simulink model "VB_RIFKF_UWB_INS25"  (R2023a)
settings: Solver=FixedStepAuto  StartTime=0.0  StopTime=500  FixedStep=0.01  RelTol=1e-3
InitFcn:
  | resilient_initNavigation1216;
  | init_param;
  | param_bias;
undefined symbols (not defined in the file or in its folder): dt, g0, gam0_rad, ISUS_flag, lp_GPS_sample_time, lp_Lidar_knoise, lp_Lidar_max, lp_Lidar_min, lp_Lidar_sample_time, lp_Lidar_seed, lp_UWB_knoise, lp_UWB_sample_time, lp_UWB_seed, lp_UWB_XY_max, lp_UWB_XY_min, magnitude, p, P0, P0_RIEKF, param, pd0, pe0, phi0_rad, pn0, psi, psi0_rad, state_dim, vd0, ve0, vn0
libraries: simulink_extras x108, simulink x89, dspstat3 x74, sharedtransform x61, matrix_library x11, sharedTrackingLibrary x8, aerolibconvert2 x5, aerolibtransform2 x5, dspfactors x3
(part 2 of 29)

== system VB_RIFKF_UWB_INS25/read FC1_zy ==
  Bus Creator : BusCreator  Inputs=3
  Bus Creator1 : BusCreator  Inputs=3
  Bus Creator2 : BusCreator  Inputs=3
  Degrees to Radians : simulink_extras/Transformations/Degrees to Radians
  Degrees to Radians1 : simulink_extras/Transformations/Degrees to Radians
  Degrees to Radians2 : simulink_extras/Transformations/Degrees to Radians
  From Workspace1 : FromWorkspace  VariableName=[time(1:(end-1)),FCS1.data_tj_st.Vn(1:(end-1))]
  From Workspace10 : FromWorkspace  VariableName=[time(1:(end-1)),FCS1.data_tj_st.Ve(1:(end-1))]
  From Workspace11 : FromWorkspace  VariableName=[time(1:(end-1)),FCS1.data_tj_st.Vu(1:(end-1))]
  From Workspace12 : FromWorkspace  VariableName=[time(1:(end-1)),FCS1.data_zy_st.gy(1:(end-1))]
  From Workspace13 : FromWorkspace  VariableName=[time(1:(end-1)),FCS1.data_zy_st.gz(1:(end-1))]
  From Workspace14 : FromWorkspace  VariableName=[time(1:(end-1)),FCS1.data_zy_st.Ax(1:(end-1))]
  From Workspace15 : FromWorkspace  VariableName=[time(1:(end-1)),FCS1.data_zy_st.Ay(1:(end-1))]
  From Workspace16 : FromWorkspace  VariableName=[time(1:(end-1)),FCS1.data_zy_st.Az(1:(end-1))]
  From Workspace17 : FromWorkspace  VariableName=[time(1:(end-1)),FCS1.data_zy_st.roll(1:(end-1))]
  From Workspace18 : FromWorkspace  VariableName=[time(1:(end-1)),FCS1.data_zy_st.pitch(1:(end-1))]
  From Workspace19 : FromWorkspace  VariableName=[time(1:(end-1)),FCS1.data_zy_st.yaw(1:(end-1))]
  From Workspace2 : FromWorkspace  VariableName=[time(1:(end-1)),FCS1.data_zy_st.gx(1:(end-1))]
  From Workspace7 : FromWorkspace  VariableName=[time(1:(end-1)),FCS1.data_zy_st.lat(1:(end-1))]
  From Workspace8 : FromWorkspace  VariableName=[time(1:(end-1)),FCS1.data_zy_st.lon(1:(end-1))]
  From Workspace9 : FromWorkspace  VariableName=[time(1:(end-1)),FCS1.data_zy_st.height(1:(end-1))]
  Gain1 : Gain  Gain=-1
  MATLAB Function : MATLAB Function  TreatAsAtomicUnit=on
  Mux : Mux  Inputs=3
  Mux2 : Mux  Inputs=3
  Mux3 : Mux  Inputs=3
  Scope{,2,4..9} (8 alike) : Scope
  Subsystem : Subsystem
  Subsystem1 : Subsystem
  Subsystem2 : Subsystem
  Zero-Order Hold9 : ZeroOrderHold  SampleTime=dt
  vned_GPS : Outport
  GPS_lla_rad : Outport  Port=2
  wxyz : Outport  Port=3
  fbxyz : Outport  Port=4
  magn : Outport  Port=5
  att_ref : Outport  Port=6
  wires:
  Mux3/1 -> Zero-Order Hold9/1
  From Workspace17/1 -> Bus Creator2/1  "roll"
  From Workspace19/1 -> MATLAB Function/1(dpsi)
  From Workspace11/1 -> Gain1/1
  Bus Creator2/1 -> Scope9/1, att_ref/1, Scope8/1
  Degrees to Radians2/1 -> wxyz/1, Scope6/1
  From Workspace15/1 -> Bus Creator1/2
  Subsystem/1(y) -> Bus Creator/1
  From Workspace14/1 -> Bus Creator1/1
  Zero-Order Hold9/1 -> magn/1
  Degrees to Radians1/1 -> Mux2/2
  Subsystem2/1(y) -> Bus Creator/3
  MATLAB Function/1(y) -> Bus Creator2/3  "yaw"
  From Workspace1/1 -> Mux/1  "vn"
  From Workspace9/1 -> Mux2/3  "altitude"
  Mux/1 -> Scope2/1, vned_GPS/1
  From Workspace16/1 -> Bus Creator1/3
  From Workspace12/1 -> Scope7/1, Subsystem1/1(u)
  From Workspace8/1 -> Degrees to Radians1/1  "lon"
  Bus Creator/1 -> Scope4/1, Degrees to Radians2/1
  Bus Creator1/1 -> fbxyz/1, Scope5/1
  Mux2/1 -> GPS_lla_rad/1, Scope/1
  Gain1/1 -> Mux/3
  From Workspace18/1 -> Bus Creator2/2  "pitch"
  From Workspace10/1 -> Mux/2  "ve"
  Degrees to Radians/1 -> Mux2/1
  Subsystem1/1(y) -> Bus Creator/2
  From Workspace7/1 -> Degrees to Radians/1  "lat"
  From Workspace2/1 -> Subsystem/1(u)
  From Workspace13/1 -> Subsystem2/1(u)

== system VB_RIFKF_UWB_INS25/read FC1_zy1 ==
  Bus Creator2 : BusCreator  Inputs=3
  Degrees to Radians : simulink_extras/Transformations/Degrees to Radians
  Degrees to Radians1 : simulink_extras/Transformations/Degrees to Radians
  From Workspace1 : FromWorkspace  VariableName=[time(1:(end-1)),FCS1.data_tj_st.Vn(1:(end-1))]
  From Workspace10 : FromWorkspace  VariableName=[time(1:(end-1)),FCS1.data_tj_st.Ve(1:(end-1))]
  From Workspace11 : FromWorkspace  VariableName=[time(1:(end-1)),FCS1.data_tj_st.Vu(1:(end-1))]
  From Workspace17 : FromWorkspace  VariableName=[time(1:(end-1)),FCS1.data_zy_st.roll(1:(end-1))]
  From Workspace18 : FromWorkspace  VariableName=[time(1:(end-1)),FCS1.data_zy_st.pitch(1:(end-1))]
  From Workspace19 : FromWorkspace  VariableName=[time(1:(end-1)),FCS1.data_zy_st.yaw(1:(end-1))]
  From Workspace7 : FromWorkspace  VariableName=[time(1:(end-1)),FCS1.data_tj_st.lat(1:(end-1))]
  From Workspace8 : FromWorkspace  VariableName=[time(1:(end-1)),FCS1.data_tj_st.lon(1:(end-1))]
  From Workspace9 : FromWorkspace  VariableName=[time(1:(end-1)),FCS1.data_tj_st.height(1:(end-1))]
  Gain1 : Gain  Gain=-1
  MATLAB Function : MATLAB Function  TreatAsAtomicUnit=on
  Mux : Mux  Inputs=3
  Mux2 : Mux  Inputs=3
  Mux3 : Mux  Inputs=3
  Scope{,2,8..9} (4 alike) : Scope
  Zero-Order Hold9 : ZeroOrderHold  SampleTime=dt
  vned_GPS : Outport
  GPS_lla_rad : Outport  Port=2
  magn : Outport  Port=3
  att_ref : Outport  Port=4
  wires:
  From Workspace7/1 -> Degrees to Radians/1  "lat"
  Degrees to Radians/1 -> Mux2/1
  From Workspace10/1 -> Mux/2  "ve"
  From Workspace18/1 -> Bus Creator2/2  "pitch"
  Gain1/1 -> Mux/3
  Mux2/1 -> Scope/1, GPS_lla_rad/1
  From Workspace8/1 -> Degrees to Radians1/1  "lon"
  Mux/1 -> vned_GPS/1, Scope2/1
  From Workspace9/1 -> Mux2/3  "altitude"
  From Workspace1/1 -> Mux/1  "vn"
  MATLAB Function/1(y) -> Bus Creator2/3  "yaw"
  Degrees to Radians1/1 -> Mux2/2
  Zero-Order Hold9/1 -> magn/1
  Bus Creator2/1 -> Scope8/1, att_ref/1, Scope9/1
  From Workspace11/1 -> Gain1/1
  From Workspace19/1 -> MATLAB Function/1(dpsi)
  From Workspace17/1 -> Bus Creator2/1  "roll"
  Mux3/1 -> Zero-Order Hold9/1

== system VB_RIFKF_UWB_INS25/read FC6_zy2 ==
  Bus Creator : BusCreator  Inputs=3
  Bus Creator1 : BusCreator  Inputs=3
  Bus Creator2 : BusCreator  Inputs=3
  Degrees to Radians : simulink_extras/Transformations/Degrees to Radians
  Degrees to Radians1 : simulink_extras/Transformations/Degrees to Radians
  Degrees to Radians2 : simulink_extras/Transformations/Degrees to Radians
  From Workspace1 : FromWorkspace  VariableName=[time1(1:(end-1)),FCS6.data_zy_st.Vn(1:(end-1))]
  From Workspace10 : FromWorkspace  VariableName=[time1(1:(end-1)),FCS6.data_zy_st.Ve(1:(end-1))]
  From Workspace11 : FromWorkspace  VariableName=[time1(1:(end-1)),FCS6.data_zy_st.Vu(1:(end-1))]
  From Workspace12 : FromWorkspace  VariableName=[time1(1:(end-1)),FCS6.data_hf_st.gy(1:(end-1))]
  From Workspace13 : FromWorkspace  VariableName=[time1(1:(end-1)),FCS6.data_hf_st.gz(1:(end-1))]
  From Workspace14 : FromWorkspace  VariableName=[time1(1:(end-1)),FCS6.data_hf_st.Ax(1:(end-1))]
  From Workspace15 : FromWorkspace  VariableName=[time1(1:(end-1)),FCS6.data_hf_st.Ay(1:(end-1))]
  From Workspace16 : FromWorkspace  VariableName=[time1(1:(end-1)),FCS6.data_hf_st.Az(1:(end-1))]
  From Workspace17 : FromWorkspace  VariableName=[time1(1:(end-1)),FCS6.data_zy_st.roll(1:(end-1))]
  From Workspace18 : FromWorkspace  VariableName=[time1(1:(end-1)),FCS6.data_zy_st.pitch(1:(end-1))]
  From Workspace19 : FromWorkspace  VariableName=[time1(1:(end-1)),FCS6.data_zy_st.yaw(1:(end-1))]
  From Workspace2 : FromWorkspace  VariableName=[time1(1:(end-1)),FCS6.data_hf_st.gx(1:(end-1))]
  From Workspace7 : FromWorkspace  VariableName=[time1(1:(end-1)),FCS6.data_zy_st.lat(1:(end-1))]
  From Workspace8 : FromWorkspace  VariableName=[time1(1:(end-1)),FCS6.data_zy_st.lon(1:(end-1))]
  From Workspace9 : FromWorkspace  VariableName=[time1(1:(end-1)),FCS6.data_zy_st.height(1:(end-1))]
  Gain1 : Gain  Gain=-1
  MATLAB Function : MATLAB Function  TreatAsAtomicUnit=on
  Mux : Mux  Inputs=3
  Mux2 : Mux  Inputs=3
  Mux3 : Mux  Inputs=3
  Scope{,2,4..6,8..9} (7 alike) : Scope
  Subsystem : Subsystem
  Subsystem1 : Subsystem
  Subsystem2 : Subsystem
  Zero-Order Hold9 : ZeroOrderHold  SampleTime=dt
  wxyz : Outport
  fbxyz : Outport  Port=2
  vned_GPS : Outport  Port=3
  GPS_lla_rad : Outport  Port=4
  magn : Outport  Port=5
  att_ref : Outport  Port=6
  wires:
  Mux3/1 -> Zero-Order Hold9/1
  From Workspace17/1 -> Bus Creator2/1  "roll"
  From Workspace19/1 -> MATLAB Function/1(dpsi)
  From Workspace11/1 -> Gain1/1
  Bus Creator2/1 -> Scope9/1, att_ref/1, Scope8/1
  Zero-Order Hold9/1 -> magn/1
  Degrees to Radians1/1 -> Mux2/2
  MATLAB Function/1(y) -> Bus Creator2/3  "yaw"
  From Workspace1/1 -> Mux/1  "vn"
  From Workspace9/1 -> Mux2/3  "altitude"
  Mux/1 -> Scope2/1, vned_GPS/1
  From Workspace8/1 -> Degrees to Radians1/1  "lon"
  Mux2/1 -> GPS_lla_rad/1, Scope/1
  Gain1/1 -> Mux/3
  From Workspace18/1 -> Bus Creator2/2  "pitch"
  From Workspace10/1 -> Mux/2  "ve"
  Degrees to Radians/1 -> Mux2/1
  From Workspace7/1 -> Degrees to Radians/1  "lat"
  From Workspace2/1 -> Subsystem/1(u)
  Subsystem1/1(y) -> Bus Creator/2
  From Workspace13/1 -> Subsystem2/1(u)
  Bus Creator1/1 -> fbxyz/1, Scope5/1
  Degrees to Radians2/1 -> wxyz/1, Scope6/1
  Subsystem2/1(y) -> Bus Creator/3
  From Workspace15/1 -> Bus Creator1/2
  Subsystem/1(y) -> Bus Creator/1
  From Workspace16/1 -> Bus Creator1/3
  Bus Creator/1 -> Scope4/1, Degrees to Radians2/1
  From Workspace12/1 -> Subsystem1/1(u)
  From Workspace14/1 -> Bus Creator1/1

== system VB_RIFKF_UWB_INS25/相对传感器模拟1 ==
  #2P : Inport
  #1GPS1 : Inport  Port=2
  Add : Sum  Inputs=-+
  Add2 : Sum  Inputs=+-
  Atan1 : Trigonometry  Operator=atan2
  Atan3 : Trigonometry  Operator=cos
  Atan4 : Trigonometry
  Bus Creator : BusCreator  Inputs=5
  Bus Selector : BusSelector  OutputSignals=GPS_Data.pos_N_gps,GPS_Data.pos_E_gps,GPS_Data.pos_D_gps
  Bus Selector1 : BusSelector  OutputSignals=GPS_Data.pos_N_gps,GPS_Data.pos_E_gps,GPS_Data.pos_D_gps
  Delay : Delay  DelayLength=1
  Delay1 : Delay  DelayLength=1
  Delay2 : Delay  DelayLength=1
  Display : Display
  Display2 : Display
  Display3 : Display
  Dot Product : DotProduct  OutDataTypeStr=Inherit: Inherit via internal rule
  MATLAB Function : MATLAB Function  Commented=on  TreatAsAtomicUnit=on
  Mux : Mux  Inputs=2
  Mux1 : Mux  Inputs=3
  Mux2 : Mux  Inputs=2
  Mux3 : Mux  Inputs=3
  Radians to Degrees1 : simulink_extras/Transformations/Radians to Degrees
  Radians to Degrees2 : simulink_extras/Transformations/Radians to Degrees
  Radians to Degrees3 : simulink_extras/Transformations/Radians to Degrees
  Scope{,1..2,4,6..9} (8 alike) : Scope
  Scope10 : Scope  NumInputPorts=2
  Sqrt3 : Sqrt
  Subsystem : Subsystem
  Subsystem2 : Subsystem
  Sum of Elements : Sum  Inputs=+
  delta_x : Selector  InputPortWidth=3  IndexOptions=Index vector (dialog)  Indices=[1]  OutputSizes=1
  delta_x2 : Selector  InputPortWidth=3  IndexOptions=Index vector (dialog)  Indices=[1 2]  OutputSizes=1
  delta_y : Selector  InputPortWidth=3  IndexOptions=Index vector (dialog)  Indices=[2]  OutputSizes=1
  p_r_psi_phi : Outport
  wires:
  #1GPS1/1 -> Bus Selector/1
  Delay2/1 -> Bus Creator/4  "p2_k-1"
  Delay1/1 -> Mux2/2
  Delay/1 -> Mux/2
  #2P/1 -> Bus Selector1/1  "p2"
  Bus Selector1/3 -> Mux3/3  "<pos_D_gps>"
  Bus Selector1/2 -> Mux3/2  "<pos_E_gps>"
  Bus Selector1/1 -> Mux3/1  "<pos_N_gps>"
  Bus Selector/3 -> Mux1/3  "<pos_D_gps>"
  Bus Selector/2 -> Mux1/2  "<pos_E_gps>"
  Bus Selector/1 -> Mux1/1  "<pos_N_gps>"
  Add2/1 -> Scope8/1
  Atan1/1 -> Mux/1, Atan3/1, Atan4/1, Radians to Degrees2/1, Delay/1
  Mux3/1 -> Add/2, Scope10/2, Bus Creator/3, Delay2/1  "p2"
  Atan4/1 -> Scope7/1
  Atan3/1 -> Scope6/1
  MATLAB Function/1(y) -> Radians to Degrees3/1
  Radians to Degrees3/1 -> Scope2/1
  delta_x2/1 -> Dot Product/2, Dot Product/1
  Radians to Degrees1/1 -> Scope1/1, Add2/2
  Mux1/1 -> Add/1, Scope10/1
  delta_x/1 -> Display3/1, MATLAB Function/2(dx), Atan1/2
  delta_y/1 -> Display2/1, MATLAB Function/1(dy), Atan1/1
  Mux/1 -> Subsystem/1("psi ")
  Mux2/1 -> Subsystem2/1(r_xyz)
  Sum of Elements/1 -> Sqrt3/1
  Dot Product/1 -> Sum of Elements/1
  Sqrt3/1 -> Mux2/1, Scope4/1, Delay1/1, Display/1  "r12"
  Subsystem2/1(r_xyz out) -> Bus Creator/2  "r"
  Add/1 -> delta_x2/1, delta_x/1, delta_y/1, Bus Creator/5, Scope9/1  "dp"
  Subsystem/1(psi  out) -> Bus Creator/1  "psi"
  Bus Creator/1 -> p_r_psi_phi/1
  Radians to Degrees2/1 -> Scope/1, Add2/1

== system VB_RIFKF_UWB_INS25/相对传感器模拟2 ==
  #2P : Inport
  #1GPS1 : Inport  Port=2
  #1GPS2 : Inport  Port=3
  Add : Sum  Inputs=-+
  Add2 : Sum  Inputs=+-
  Atan1 : Trigonometry  Operator=atan2
  Atan3 : Trigonometry  Operator=cos
  Atan4 : Trigonometry
  Bus Creator : BusCreator  Inputs=5
  Bus Selector : BusSelector  OutputSignals=GPS_Data.pos_N_gps,GPS_Data.pos_E_gps,GPS_Data.pos_D_gps
  Bus Selector1 : BusSelector  OutputSignals=GPS_Data.pos_N_gps,GPS_Data.pos_E_gps,GPS_Data.pos_D_gps
  Delay : Delay  DelayLength=1
  Delay1 : Delay  DelayLength=1
  Delay2 : Delay  DelayLength=1
  Digital Clock : DigitalClock  SampleTime=0.01
  Display : Display
  Display2 : Display
  Display3 : Display
  Dot Product : DotProduct  OutDataTypeStr=Inherit: Inherit via internal rule
  MATLAB Function : MATLAB Function  Commented=on  TreatAsAtomicUnit=on
  Mux : Mux  Inputs=2
  Mux1 : Mux  Inputs=3
  Mux2 : Mux  Inputs=2
  Mux3 : Mux  Inputs=3
  Radians to Degrees1 : simulink_extras/Transformations/Radians to Degrees
  Radians to Degrees2 : simulink_extras/Transformations/Radians to Degrees
  Radians to Degrees3 : simulink_extras/Transformations/Radians to Degrees
  Scope{,1..2,4,6..9} (8 alike) : Scope
  Scope10 : Scope  NumInputPorts=2
  Sqrt3 : Sqrt
  Subsystem : Subsystem
  Subsystem2 : Subsystem
  Sum of Elements : Sum  Inputs=+
  Switch2 : Switch  Criteria=u2 > Threshold  Threshold=300  SaturateOnIntegerOverflow=off  InputSameDT=off
  delta_x : Selector  InputPortWidth=3  IndexOptions=Index vector (dialog)  Indices=[1]  OutputSizes=1
  delta_x2 : Selector  InputPortWidth=3  IndexOptions=Index vector (dialog)  Indices=[1 2]  OutputSizes=1
  delta_y : Selector  InputPortWidth=3  IndexOptions=Index vector (dialog)  Indices=[2]  OutputSizes=1
  p_r_psi_phi : Outport
  wires:
  Radians to Degrees2/1 -> Add2/1, Scope/1
  Bus Creator/1 -> p_r_psi_phi/1
  Subsystem/1(psi  out) -> Bus Creator/1  "psi"
  Add/1 -> Scope9/1, Bus Creator/5, delta_y/1, delta_x/1, delta_x2/1  "dp"
  Subsystem2/1(r_xyz out) -> Bus Creator/2  "r"
  Sqrt3/1 -> Display/1, Delay1/1, Scope4/1, Mux2/1  "r12"
  Dot Product/1 -> Sum of Elements/1
  Sum of Elements/1 -> Sqrt3/1
  Mux2/1 -> Subsystem2/1(r_xyz)
  Mux/1 -> Subsystem/1("psi ")
  delta_y/1 -> Atan1/1, MATLAB Function/1(dy), Display2/1
  delta_x/1 -> Atan1/2, MATLAB Function/2(dx), Display3/1
  Mux1/1 -> Scope10/1, Add/1
  Radians to Degrees1/1 -> Add2/2, Scope1/1
  delta_x2/1 -> Dot Product/1, Dot Product/2
  Radians to Degrees3/1 -> Scope2/1
  MATLAB Function/1(y) -> Radians to Degrees3/1
  Atan3/1 -> Scope6/1
  Atan4/1 -> Scope7/1
  Mux3/1 -> Delay2/1, Bus Creator/3, Scope10/2, Add/2  "p2"
  Atan1/1 -> Delay/1, Radians to Degrees2/1, Atan4/1, Atan3/1, Mux/1
  Add2/1 -> Scope8/1
  #1GPS1/1 -> Switch2/3
  Bus Selector/1 -> Mux1/1  "<pos_N_gps>"
  Bus Selector/2 -> Mux1/2  "<pos_E_gps>"
  Bus Selector/3 -> Mux1/3  "<pos_D_gps>"
  Bus Selector1/1 -> Mux3/1  "<pos_N_gps>"
  Bus Selector1/2 -> Mux3/2  "<pos_E_gps>"
  Bus Selector1/3 -> Mux3/3  "<pos_D_gps>"
  #2P/1 -> Bus Selector1/1  "p2"
  Delay/1 -> Mux/2
  Delay1/1 -> Mux2/2
  Delay2/1 -> Bus Creator/4  "p2_k-1"
  Digital Clock/1 -> Switch2/2
  #1GPS2/1 -> Switch2/1
  Switch2/1 -> Bus Selector/1

== system VB_RIFKF_UWB_INS25/相对传感器模拟3 ==
  #2P : Inport
  #1GPS2 : Inport  Port=2
  Add : Sum  Inputs=-+
  Add2 : Sum  Inputs=+-
  Atan1 : Trigonometry  Operator=atan2
  Atan3 : Trigonometry  Operator=cos
  Atan4 : Trigonometry
  Bus Creator : BusCreator  Inputs=5
  Bus Selector : BusSelector  OutputSignals=GPS_Data.pos_N_gps,GPS_Data.pos_E_gps,GPS_Data.pos_D_gps
  Bus Selector1 : BusSelector  OutputSignals=GPS_Data.pos_N_gps,GPS_Data.pos_E_gps,GPS_Data.pos_D_gps
  Delay : Delay  DelayLength=1
  Delay1 : Delay  DelayLength=1
  Delay2 : Delay  DelayLength=1
  Display : Display
  Display2 : Display
  Display3 : Display
  Dot Product : DotProduct  OutDataTypeStr=Inherit: Inherit via internal rule
  MATLAB Function : MATLAB Function  Commented=on  TreatAsAtomicUnit=on
  Mux : Mux  Inputs=2
  Mux1 : Mux  Inputs=3
  Mux2 : Mux  Inputs=2
  Mux3 : Mux  Inputs=3
  Radians to Degrees1 : simulink_extras/Transformations/Radians to Degrees
  Radians to Degrees2 : simulink_extras/Transformations/Radians to Degrees
  Radians to Degrees3 : simulink_extras/Transformations/Radians to Degrees
  Scope{,1..2,4,6..9} (8 alike) : Scope
  Scope10 : Scope  NumInputPorts=2
  Sqrt3 : Sqrt
  Subsystem : Subsystem
  Subsystem2 : Subsystem
  Sum of Elements : Sum  Inputs=+
  delta_x : Selector  InputPortWidth=3  IndexOptions=Index vector (dialog)  Indices=[1]  OutputSizes=1
  delta_x2 : Selector  InputPortWidth=3  IndexOptions=Index vector (dialog)  Indices=[1 2]  OutputSizes=1
  delta_y : Selector  InputPortWidth=3  IndexOptions=Index vector (dialog)  Indices=[2]  OutputSizes=1
  p_r_psi_phi : Outport
  wires:
  Radians to Degrees2/1 -> Add2/1, Scope/1
  Bus Creator/1 -> p_r_psi_phi/1
  Subsystem/1(psi  out) -> Bus Creator/1  "psi"
  Add/1 -> Scope9/1, Bus Creator/5, delta_y/1, delta_x/1, delta_x2/1  "dp"
  Subsystem2/1(r_xyz out) -> Bus Creator/2  "r"
  Sqrt3/1 -> Display/1, Delay1/1, Scope4/1, Mux2/1  "r12"
  Dot Product/1 -> Sum of Elements/1
  Sum of Elements/1 -> Sqrt3/1
  Mux2/1 -> Subsystem2/1(r_xyz)
  Mux/1 -> Subsystem/1("psi ")
  delta_y/1 -> Atan1/1, MATLAB Function/1(dy), Display2/1
  delta_x/1 -> Atan1/2, MATLAB Function/2(dx), Display3/1
  Mux1/1 -> Scope10/1, Add/1
  Radians to Degrees1/1 -> Add2/2, Scope1/1
  delta_x2/1 -> Dot Product/1, Dot Product/2
  Radians to Degrees3/1 -> Scope2/1
  MATLAB Function/1(y) -> Radians to Degrees3/1
  Atan3/1 -> Scope6/1
  Atan4/1 -> Scope7/1
  Mux3/1 -> Delay2/1, Bus Creator/3, Scope10/2, Add/2  "p2"
  Atan1/1 -> Delay/1, Radians to Degrees2/1, Atan4/1, Atan3/1, Mux/1
  Add2/1 -> Scope8/1
  Bus Selector/1 -> Mux1/1  "<pos_N_gps>"
  Bus Selector/2 -> Mux1/2  "<pos_E_gps>"
  Bus Selector/3 -> Mux1/3  "<pos_D_gps>"
  Bus Selector1/1 -> Mux3/1  "<pos_N_gps>"
  Bus Selector1/2 -> Mux3/2  "<pos_E_gps>"
  Bus Selector1/3 -> Mux3/3  "<pos_D_gps>"
  #2P/1 -> Bus Selector1/1  "p2"
  Delay/1 -> Mux/2
  Delay1/1 -> Mux2/2
  Delay2/1 -> Bus Creator/4  "p2_k-1"
  #1GPS2/1 -> Bus Selector/1

== system VB_RIFKF_UWB_INS25/相对传感器模拟4 ==
  #2P : Inport
  #1GPS3 : Inport  Port=2
  Add : Sum  Inputs=-+
  Add2 : Sum  Inputs=+-
  Atan1 : Trigonometry  Operator=atan2
  Atan3 : Trigonometry  Operator=cos
  Atan4 : Trigonometry
  Bus Creator : BusCreator  Inputs=5
  Bus Selector : BusSelector  OutputSignals=GPS_Data.pos_N_gps,GPS_Data.pos_E_gps,GPS_Data.pos_D_gps
  Bus Selector1 : BusSelector  OutputSignals=GPS_Data.pos_N_gps,GPS_Data.pos_E_gps,GPS_Data.pos_D_gps
  Delay : Delay  DelayLength=1
  Delay1 : Delay  DelayLength=1
  Delay2 : Delay  DelayLength=1
  Display : Display
  Display2 : Display
  Display3 : Display
  Dot Product : DotProduct  OutDataTypeStr=Inherit: Inherit via internal rule
  MATLAB Function : MATLAB Function  Commented=on  TreatAsAtomicUnit=on
  Mux : Mux  Inputs=2
  Mux1 : Mux  Inputs=3
  Mux2 : Mux  Inputs=2
  Mux3 : Mux  Inputs=3
  Radians to Degrees1 : simulink_extras/Transformations/Radians to Degrees
  Radians to Degrees2 : simulink_extras/Transformations/Radians to Degrees
  Radians to Degrees3 : simulink_extras/Transformations/Radians to Degrees
  Scope{,1..2,4,6..9} (8 alike) : Scope
  Scope10 : Scope  NumInputPorts=2
  Sqrt3 : Sqrt
  Subsystem : Subsystem
  Subsystem2 : Subsystem
  Sum of Elements : Sum  Inputs=+
  delta_x : Selector  InputPortWidth=3  IndexOptions=Index vector (dialog)  Indices=[1]  OutputSizes=1
  delta_x2 : Selector  InputPortWidth=3  IndexOptions=Index vector (dialog)  Indices=[1 2]  OutputSizes=1
  delta_y : Selector  InputPortWidth=3  IndexOptions=Index vector (dialog)  Indices=[2]  OutputSizes=1
  p_r_psi_phi : Outport
  wires:
  #1GPS3/1 -> Bus Selector/1
  Delay2/1 -> Bus Creator/4  "p2_k-1"
  Delay1/1 -> Mux2/2
  Delay/1 -> Mux/2
  #2P/1 -> Bus Selector1/1  "p2"
  Bus Selector1/3 -> Mux3/3  "<pos_D_gps>"
  Bus Selector1/2 -> Mux3/2  "<pos_E_gps>"
  Bus Selector1/1 -> Mux3/1  "<pos_N_gps>"
  Bus Selector/3 -> Mux1/3  "<pos_D_gps>"
  Bus Selector/2 -> Mux1/2  "<pos_E_gps>"
  Bus Selector/1 -> Mux1/1  "<pos_N_gps>"
  Add2/1 -> Scope8/1
  Atan1/1 -> Mux/1, Atan3/1, Atan4/1, Radians to Degrees2/1, Delay/1
  Mux3/1 -> Add/2, Scope10/2, Bus Creator/3, Delay2/1  "p2"
  Atan4/1 -> Scope7/1
  Atan3/1 -> Scope6/1
  MATLAB Function/1(y) -> Radians to Degrees3/1
  Radians to Degrees3/1 -> Scope2/1
  delta_x2/1 -> Dot Product/2, Dot Product/1
  Radians to Degrees1/1 -> Scope1/1, Add2/2
  Mux1/1 -> Add/1, Scope10/1
  delta_x/1 -> Display3/1, MATLAB Function/2(dx), Atan1/2
  delta_y/1 -> Display2/1, MATLAB Function/1(dy), Atan1/1
  Mux/1 -> Subsystem/1("psi ")
  Mux2/1 -> Subsystem2/1(r_xyz)
  Sum of Elements/1 -> Sqrt3/1
  Dot Product/1 -> Sum of Elements/1
  Sqrt3/1 -> Mux2/1, Scope4/1, Delay1/1, Display/1  "r12"
  Subsystem2/1(r_xyz out) -> Bus Creator/2  "r"
  Add/1 -> delta_x2/1, delta_x/1, delta_y/1, Bus Creator/5, Scope9/1  "dp"
  Subsystem/1(psi  out) -> Bus Creator/1  "psi"
  Bus Creator/1 -> p_r_psi_phi/1
  Radians to Degrees2/1 -> Scope/1, Add2/1

== system VB_RIFKF_UWB_INS25/ER EKF M1/Bus_Constructor ==
  INSstate : Inport
  Bus Creator : BusCreator  Inputs=2
  Bus Creator1 : BusCreator  Inputs=2
  Bus Creator3 : BusCreator  Inputs=6
  Bus Selector : BusSelector  OutputSignals=RotationData.q_update,RotationData.DCM_b_n,INSstate_v,INSstste_p,INSstate_dg,INSstate_da
  Demux2 : Demux  Outputs=3
  Demux3 : Demux  Outputs=3
  Scope : Scope
  TranslationData : Outport
  RotationData : Outport  Port=2
  INSbiasData : Outport  Port=3
  wires:
  INSstate/1 -> Bus Selector/1
  Bus Selector/2 -> Bus Creator/2  "<DCM_b_n>"
  Bus Selector/1 -> Bus Creator/1  "<q_update>"
  Bus Creator/1 -> RotationData/1
  Bus Selector/5 -> Bus Creator1/1  "<INSstate_dg>"
  Bus Selector/6 -> Bus Creator1/2  "<INSstate_da>"
  Bus Creator1/1 -> INSbiasData/1
  Demux2/3 -> Bus Creator3/3  "vd_m/s"
  Demux2/1 -> Bus Creator3/1  "vn_m/s"
  Demux3/3 -> Bus Creator3/6  "pd_m"
  Demux3/1 -> Bus Creator3/4  "pn_m"
  Bus Creator3/1 -> Scope/1, TranslationData/1
  Demux2/2 -> Bus Creator3/2  "ve_m/s"
  Demux3/2 -> Bus Creator3/5  "pe_m"
  Bus Selector/3 -> Demux2/1  "<INSstate_v>"
  Bus Selector/4 -> Demux3/1  "<INSstste_p>"

== system VB_RIFKF_UWB_INS25/ER EKF M1/Bus_Constructor2 ==
  TranlationData : Inport
  RotationData : Inport  Port=2
  INSbiasData : Inport  Port=3
  GNSS enable flag : Inport  Port=4
  Bus Creator : BusCreator  Inputs=4
  Rotation_output : Subsystem
  Scope : Scope
  RI EKFNav_out : Outport
  wires:
  GNSS enable flag/1 -> Bus Creator/4  "GNSS enable flag"
  RotationData/1 -> Rotation_output/1(RotationData)  "RotationData"
  Bus Creator/1 -> RI EKFNav_out/1
  TranlationData/1 -> Bus Creator/1  "TranlationData"
  Rotation_output/1(psi_theta_phi_rad) -> Scope/1, Bus Creator/2  "RotationData"
  INSbiasData/1 -> Bus Creator/3  "INSbiasData"

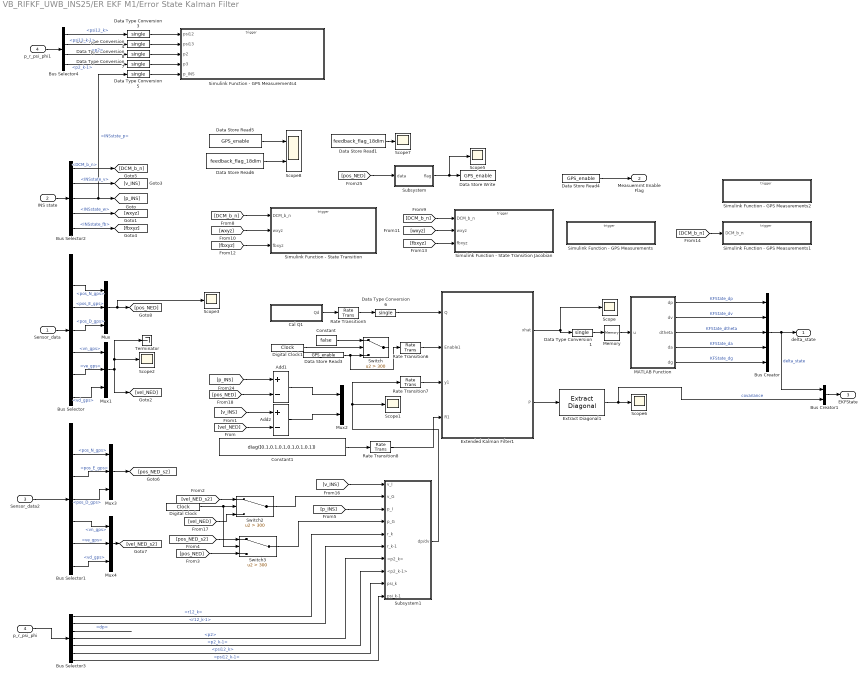
== system VB_RIFKF_UWB_INS25/ER EKF M1/Error State Kalman Filter ==
  Sensor_data : Inport
  INS state : Inport  Port=2
  Sensor_data2 : Inport  Port=3
  p_r_psi_phi : Inport  Port=4
  Add1 : Sum  Inputs=+-
  Add2 : Sum  Inputs=+-
  Bus Creator : BusCreator  Inputs=5
  Bus Creator1 : BusCreator  Inputs=2
  Bus Selector : BusSelector  OutputSignals=QGC_sensor_reinit,GPS_Data.pos_N_gps,GPS_Data.pos_E_gps,GPS_Data.pos_D_gps,GPS_Data.vn_gps,GPS_Data.ve_gps,GPS_Data.vd_gps
  Bus Selector1 : BusSelector  OutputSignals=QGC_sensor_reinit,GPS_Data.pos_N_gps,GPS_Data.pos_E_gps,GPS_Data.pos_D_gps,GPS_Data.vn_gps,GPS_Data.ve_gps,GPS_Data.vd_gps
  Bus Selector2 : BusSelector  OutputSignals=RotationData.DCM_b_n,INSstate_v,INSstste_p,INSstate_w,INSstate_fb
  Bus Selector3 : BusSelector  OutputSignals=r.r12_k,r.r12_k-1,dp,p2,p2_k-1,psi.psi12_k,psi.psi12_k-1
  Bus Selector4 : BusSelector  OutputSignals=psi.psi12_k,psi.psi12_k-1,p2,p2_k-1
  Cal Q1 : Subsystem
  Constant : Constant  Value=false
  Constant1 : Constant  Value=diag([0.1,0.1,0.1,0.1,0.1,0.1])  OutDataTypeStr=single
  Data Store Read1 : DataStoreRead  DataStoreName=feedback_flag_18dim  IndexOptions=Index vector (dialog)  Indices=1  OutputSizes=1
  Data Store Read3 : DataStoreRead  DataStoreName=GPS_enable  IndexOptions=Index vector (dialog)  Indices=1  OutputSizes=1
  Data Store Read4 : DataStoreRead  DataStoreName=GPS_enable  IndexOptions=Index vector (dialog)  Indices=1  OutputSizes=1
  Data Store Read5 : DataStoreRead  DataStoreName=GPS_enable  IndexOptions=Index vector (dialog)  Indices=1  OutputSizes=1
  Data Store Read6 : DataStoreRead  DataStoreName=feedback_flag_18dim  IndexOptions=Index vector (dialog)  Indices=1  OutputSizes=1
  Data Store Write : DataStoreWrite  DataStoreName=GPS_enable  IndexOptions=Index vector (dialog)  Indices=1  OutputSizes=1
  Data Type Conversion{1,3..8} (7 alike) : DataTypeConversion  OutDataTypeStr=single  SaturateOnIntegerOverflow=off  RndMeth=Floor
  Digital Clock : DigitalClock  SampleTime=0.01
  Digital Clock1 : DigitalClock  SampleTime=0.01
  Extended Kalman Filter1 : Subsystem  mask(Extended Kalman Filter){StateTransitionFcn=stateTransitionFcn, HasStateTransitionJacobianFcn=on, StateTransitionJacobianFcn=stateTransitionJacobianFcn, HasAdditiveProcessNoise=Nonadditive, ProcessNoise=1, HasTimeVaryingProcessNoise=on, HasStateTransitionFcnExtraArgument=0, InitialState=zeros(15,1), InitialStateCovariance=P0, MeasurementFcn1=UWBMeasurementFcn_Dyn, HasMeasurementJacobianFcn1=off, MeasurementJacobianFcn1=, HasMeasurementEnablePort1=on, HasAdditiveMeasurementNoise1=Nonadditive, MeasurementNoise1=1, HasTimeVaryingMeasurementNoise1=on, HasMeasurementFcnExtraArgument1=0, HasMeasurementWrapping1=off, MeasurementFcn2=DynamicMeasurementFcn_Dyn, HasMeasurementJacobianFcn2=off, MeasurementJacobianFcn2=, HasMeasurementEnablePort2=on, HasAdditiveMeasurementNoise2=Nonadditive, MeasurementNoise2=1, HasTimeVaryingMeasurementNoise2=on, HasMeasurementFcnExtraArgument2=0, HasMeasurementWrapping2=off, MeasurementFcn3=ZUPTMeasurementFcn2, HasMeasurementJacobianFcn3=off, MeasurementJacobianFcn3=, HasMeasurementEnablePort3=on, HasAdditiveMeasurementNoise3=Nonadditive, MeasurementNoise3=1, HasTimeVaryingMeasurementNoise3=on, HasMeasurementFcnExtraArgument3=0, HasMeasurementWrapping3=off, MeasurementFcn4=myMeasurementFcn, HasMeasurementJacobianFcn4=off, MeasurementJacobianFcn4=, HasMeasurementEnablePort4=off, HasAdditiveMeasurementNoise4=Additive, MeasurementNoise4=1, HasTimeVaryingMeasurementNoise4=off, HasMeasurementFcnExtraArgument4=0, HasMeasurementWrapping4=off, MeasurementFcn5=myMeasurementFcn, HasMeasurementJacobianFcn5=off, MeasurementJacobianFcn5=, HasMeasurementEnablePort5=off, HasAdditiveMeasurementNoise5=Additive, MeasurementNoise5=1, HasTimeVaryingMeasurementNoise5=off, HasMeasurementFcnExtraArgument5=0, HasMeasurementWrapping5=off, EnableMultirate=off, StateTransitionFcnSampleTime=0.01, MeasurementFcn1SampleTime=0.2, MeasurementFcn2SampleTime=0.01, MeasurementFcn3SampleTime=1, MeasurementFcn4SampleTime=1, MeasurementFcn5SampleTime=1, UseCurrentEstimator=on, OutputStateCovariance=on, DataType=single, SampleTime=0.01, NumberOfMeasurements=1}
      mask prompts: HasStateTransitionJacobianFcn "shared_tracking:blocks:maskPromptEKFJacobian"; HasTimeVaryingProcessNoise "shared_tracking:blocks:maskPromptEKFUKFTimeVarying"; HasMeasurementJacobianFcn1 "shared_tracking:blocks:maskPromptEKFJacobian"; HasMeasurementEnablePort1 "shared_tracking:blocks:maskPromptEnablePort"; HasTimeVaryingMeasurementNoise1 "shared_tracking:blocks:maskPromptEKFUKFTimeVarying"; HasMeasurementWrapping1 "shared_tracking:blocks:maskPromptEKFUKFMeasurementWrapping"; HasMeasurementJacobianFcn2 "shared_tracking:blocks:maskPromptEKFJacobian"; HasMeasurementEnablePort2 "shared_tracking:blocks:maskPromptEnablePort"; HasTimeVaryingMeasurementNoise2 "shared_tracking:blocks:maskPromptEKFUKFTimeVarying"; HasMeasurementWrapping2 "shared_tracking:blocks:maskPromptEKFUKFMeasurementWrapping"; HasMeasurementJacobianFcn3 "shared_tracking:blocks:maskPromptEKFJacobian"; HasMeasurementEnablePort3 "shared_tracking:blocks:maskPromptEnablePort"; HasTimeVaryingMeasurementNoise3 "shared_tracking:blocks:maskPromptEKFUKFTimeVarying"; HasMeasurementWrapping3 "shared_tracking:blocks:maskPromptEKFUKFMeasurementWrapping"; HasMeasurementJacobianFcn4 "shared_tracking:blocks:maskPromptEKFJacobian"; HasMeasurementEnablePort4 "shared_tracking:blocks:maskPromptEnablePort"; HasTimeVaryingMeasurementNoise4 "shared_tracking:blocks:maskPromptEKFUKFTimeVarying"; HasMeasurementWrapping4 "shared_tracking:blocks:maskPromptEKFUKFMeasurementWrapping"; HasMeasurementJacobianFcn5 "shared_tracking:blocks:maskPromptEKFJacobian"; HasMeasurementEnablePort5 "shared_tracking:blocks:maskPromptEnablePort"; HasTimeVaryingMeasurementNoise5 "shared_tracking:blocks:maskPromptEKFUKFTimeVarying"; HasMeasurementWrapping5 "shared_tracking:blocks:maskPromptEKFUKFMeasurementWrapping"; EnableMultirate "shared_tracking:blocks:maskPromptEnableMultirate"; StateTransitionFcnSampleTime "shared_tracking:blocks:maskPromptStateTransition"; MeasurementFcn1SampleTime "shared_tracking:blocks:maskPromptMeasurement1"; MeasurementFcn2SampleTime "shared_tracking:blocks:maskPromptMeasurement2"; MeasurementFcn3SampleTime "shared_tracking:blocks:maskPromptMeasurement3"; MeasurementFcn4SampleTime "shared_tracking:blocks:maskPromptMeasurement4"; MeasurementFcn5SampleTime "shared_tracking:blocks:maskPromptMeasurement5"; UseCurrentEstimator "shared_tracking:blocks:maskPromptUseCurrentEstimator"; OutputStateCovariance "shared_tracking:blocks:maskPromptOutputStateCovariance"; DataType "shared_tracking:blocks:maskPromptDataType"; SampleTime "shared_tracking:blocks:maskPromptSampleTime"
      mask help: shared_tracking:blocks:maskPromptEKFDescription
      mask init:
      | matlabshared.tracking.internal.blocks.maskInitializationScriptEKF
      mask Help: eval('matlabshared.tracking.internal.blocks.controlIdentLaunchDocPage(''EKF'')')
      mask Callback HasStateTransitionJacobianFcn: matlabshared.tracking.internal.blocks.dialogCallbacksEKFUKFPF(gcbh(),'checkBoxHasJacobianFcn','StateTransition');
      mask TypeOptions HasAdditiveProcessNoise: shared_tracking:blocks:maskPromptEKFUKFAdditiveNoise | shared_tracking:blocks:maskPromptEKFUKFNonAdditiveNoise
      mask Callback HasTimeVaryingProcessNoise: matlabshared.tracking.internal.blocks.dialogCallbacksEKFUKFPF(gcbh,'checkboxIsCovarianceTimeVarying','HasTimeVaryingProcessNoise','ProcessNoise')
      mask Callback HasMeasurementJacobianFcn1: matlabshared.tracking.internal.blocks.dialogCallbacksEKFUKFPF(gcbh(),'checkBoxHasJacobianFcn','Measurement','1');
      mask TypeOptions HasAdditiveMeasurementNoise1: shared_tracking:blocks:maskPromptEKFUKFAdditiveNoise | shared_tracking:blocks:maskPromptEKFUKFNonAdditiveNoise
      mask Callback HasTimeVaryingMeasurementNoise1: matlabshared.tracking.internal.blocks.dialogCallbacksEKFUKFPF(gcbh,'checkboxIsCovarianceTimeVarying','HasTimeVaryingMeasurementNoise1','MeasurementNoise1')
      mask Callback HasMeasurementJacobianFcn2: matlabshared.tracking.internal.blocks.dialogCallbacksEKFUKFPF(gcbh(),'checkBoxHasJacobianFcn','Measurement','2');
      mask TypeOptions HasAdditiveMeasurementNoise2: shared_tracking:blocks:maskPromptEKFUKFAdditiveNoise | shared_tracking:blocks:maskPromptEKFUKFNonAdditiveNoise
      mask Callback HasTimeVaryingMeasurementNoise2: matlabshared.tracking.internal.blocks.dialogCallbacksEKFUKFPF(gcbh,'checkboxIsCovarianceTimeVarying','HasTimeVaryingMeasurementNoise2','MeasurementNoise2')
      mask Callback HasMeasurementJacobianFcn3: matlabshared.tracking.internal.blocks.dialogCallbacksEKFUKFPF(gcbh(),'checkBoxHasJacobianFcn','Measurement','3');
      mask TypeOptions HasAdditiveMeasurementNoise3: shared_tracking:blocks:maskPromptEKFUKFAdditiveNoise | shared_tracking:blocks:maskPromptEKFUKFNonAdditiveNoise
      mask Callback HasTimeVaryingMeasurementNoise3: matlabshared.tracking.internal.blocks.dialogCallbacksEKFUKFPF(gcbh,'checkboxIsCovarianceTimeVarying','HasTimeVaryingMeasurementNoise3','MeasurementNoise3')
      mask Callback HasMeasurementJacobianFcn4: matlabshared.tracking.internal.blocks.dialogCallbacksEKFUKFPF(gcbh(),'checkBoxHasJacobianFcn','Measurement','4');
      mask TypeOptions HasAdditiveMeasurementNoise4: shared_tracking:blocks:maskPromptEKFUKFAdditiveNoise | shared_tracking:blocks:maskPromptEKFUKFNonAdditiveNoise
      mask Callback HasTimeVaryingMeasurementNoise4: matlabshared.tracking.internal.blocks.dialogCallbacksEKFUKFPF(gcbh,'checkboxIsCovarianceTimeVarying','HasTimeVaryingMeasurementNoise4','MeasurementNoise4')
      mask Callback HasMeasurementJacobianFcn5: matlabshared.tracking.internal.blocks.dialogCallbacksEKFUKFPF(gcbh(),'checkBoxHasJacobianFcn','Measurement','5');
      mask TypeOptions HasAdditiveMeasurementNoise5: shared_tracking:blocks:maskPromptEKFUKFAdditiveNoise | shared_tracking:blocks:maskPromptEKFUKFNonAdditiveNoise
      mask Callback HasTimeVaryingMeasurementNoise5: matlabshared.tracking.internal.blocks.dialogCallbacksEKFUKFPF(gcbh,'checkboxIsCovarianceTimeVarying','HasTimeVaryingMeasurementNoise5','MeasurementNoise5')
      mask Callback EnableMultirate: matlabshared.tracking.internal.blocks.dialogCallbacksEKFUKFPF(gcbh,'checkBoxHasMultirate')
      mask TypeOptions DataType: shared_tracking:blocks:maskPromptDouble | shared_tracking:blocks:maskPromptSingle
      mask Callback NumberOfMeasurements: matlabshared.tracking.internal.blocks.dialogCallbacksEKFUKFPF(gcbh,'editboxNumberOfMeasurements','MeasurementFcn');
      mask DialogControl DescGroupVar Prompt: shared_tracking:blocks:maskPromptEKFTitle
      mask DialogControl TabSystemModel Prompt: shared_tracking:blocks:maskPromptSystemModel
      mask DialogControl GroupStateTransition Prompt: shared_tracking:blocks:maskPromptStateTransition
      mask DialogControl StateTransitionFunctionText Prompt: shared_tracking:blocks:maskPromptFunction
      mask DialogControl HasStateTransitionJacobianFcn Prompt: Jacobian
      mask DialogControl ProcessNoiseText Prompt: shared_tracking:blocks:maskPromptEKFUKFProcessNoise
      mask DialogControl ProcessNoiseCovarianceText Prompt: shared_tracking:blocks:maskPromptCovariance
      mask DialogControl HasTimeVaryingProcessNoise Prompt: Time-varying
      mask DialogControl InitializationContainer Prompt: shared_tracking:blocks:maskPromptInitialization
      mask DialogControl InitialStateText Prompt: shared_tracking:blocks:maskPromptEKFUKFInitialState
      mask DialogControl InitialCovarianceText Prompt: shared_tracking:blocks:maskPromptEKFUKFInitialCovariance
      mask DialogControl GroupMeasurement1 Prompt: shared_tracking:blocks:maskPromptMeasurement1
      mask DialogControl MeasurementFunction1Text Prompt: shared_tracking:blocks:maskPromptFunction
      mask DialogControl HasMeasurementJacobianFcn1 Prompt: Jacobian
      mask DialogControl HasMeasurementEnablePort1 Prompt: Add Enable port
      mask DialogControl MeasurementNoiseText1 Prompt: shared_tracking:blocks:maskPromptEKFUKFMeasurementNoise
      mask DialogControl MeasurementNoiseCovarianceText1 Prompt: shared_tracking:blocks:maskPromptCovariance
      mask DialogControl HasTimeVaryingMeasurementNoise1 Prompt: Time-varying
      mask DialogControl HasMeasurementWrapping1 Prompt: Has measurement wrapping
      mask DialogControl GroupMeasurement2 Prompt: shared_tracking:blocks:maskPromptMeasurement2
      mask DialogControl MeasurementFunction2Text Prompt: shared_tracking:blocks:maskPromptFunction
      mask DialogControl HasMeasurementJacobianFcn2 Prompt: Jacobian
      mask DialogControl HasMeasurementEnablePort2 Prompt: Add Enable port
      mask DialogControl MeasurementNoiseText2 Prompt: shared_tracking:blocks:maskPromptEKFUKFMeasurementNoise
      mask DialogControl MeasurementNoiseCovarianceText2 Prompt: shared_tracking:blocks:maskPromptCovariance
      mask DialogControl HasTimeVaryingMeasurementNoise2 Prompt: Time-varying
      mask DialogControl HasMeasurementWrapping2 Prompt: Has measurement wrapping
      mask DialogControl GroupMeasurement3 Prompt: shared_tracking:blocks:maskPromptMeasurement3
      mask DialogControl MeasurementFunction3Text Prompt: shared_tracking:blocks:maskPromptFunction
      mask DialogControl HasMeasurementJacobianFcn3 Prompt: Jacobian
      mask DialogControl HasMeasurementEnablePort3 Prompt: Add Enable port
      mask DialogControl MeasurementNoiseText3 Prompt: shared_tracking:blocks:maskPromptEKFUKFMeasurementNoise
      mask DialogControl MeasurementNoiseCovarianceText3 Prompt: shared_tracking:blocks:maskPromptCovariance
      mask DialogControl HasTimeVaryingMeasurementNoise3 Prompt: Time-varying
      mask DialogControl HasMeasurementWrapping3 Prompt: Has measurement wrapping
      mask DialogControl GroupMeasurement4 Prompt: shared_tracking:blocks:maskPromptMeasurement4
      mask DialogControl MeasurementFunction4Text Prompt: shared_tracking:blocks:maskPromptFunction
      mask DialogControl HasMeasurementJacobianFcn4 Prompt: Jacobian
      mask DialogControl HasMeasurementEnablePort4 Prompt: Add Enable port
      mask DialogControl MeasurementNoiseText4 Prompt: shared_tracking:blocks:maskPromptEKFUKFMeasurementNoise
      mask DialogControl MeasurementNoiseCovarianceText4 Prompt: shared_tracking:blocks:maskPromptCovariance
      mask DialogControl HasTimeVaryingMeasurementNoise4 Prompt: Time-varying
      mask DialogControl HasMeasurementWrapping4 Prompt: Has measurement wrapping
      mask DialogControl GroupMeasurement5 Prompt: shared_tracking:blocks:maskPromptMeasurement5
      mask DialogControl MeasurementFunction5Text Prompt: shared_tracking:blocks:maskPromptFunction
      mask DialogControl HasMeasurementJacobianFcn5 Prompt: Jacobian
      mask DialogControl HasMeasurementEnablePort5 Prompt: Add Enable port
      mask DialogControl MeasurementNoiseText5 Prompt: shared_tracking:blocks:maskPromptEKFUKFMeasurementNoise
      mask DialogControl MeasurementNoiseCovarianceText5 Prompt: shared_tracking:blocks:maskPromptCovariance
      mask DialogControl HasTimeVaryingMeasurementNoise5 Prompt: Time-varying
      mask DialogControl HasMeasurementWrapping5 Prompt: Has measurement wrapping
      mask DialogControl AddMeasurement Prompt: shared_tracking:blocks:maskPromptAddMeasurement
      mask DialogControl AddMeasurement Callback: matlabshared.tracking.internal.blocks.dialogCallbacksEKFUKFPF(gcbh,'buttonAddMeasurement','MeasurementFcn');
      mask DialogControl RemoveMeasurement Prompt: shared_tracking:blocks:maskPromptRemoveMeasurement
      mask DialogControl RemoveMeasurement Callback: matlabshared.tracking.internal.blocks.dialogCallbacksEKFUKFPF(gcbh,'buttonRemoveMeasurement','MeasurementFcn');
      mask DialogControl TabMultirate Prompt: shared_tracking:blocks:maskPromptEKFUKFMultirate
      mask DialogControl GroupMultirate Prompt: shared_tracking:blocks:maskPromptEKFUKFMultirate
      mask DialogControl EnableMultirate Prompt: Enable multirate operation
      mask DialogControl GroupMultirateSampleTimes Prompt: shared_tracking:blocks:maskPromptSampleTimeNoInheritance
      mask DialogControl StateTransitionFcnSampleTime Prompt: State Transition
      mask DialogControl MeasurementFcn1SampleTime Prompt: Measurement 1
      mask DialogControl MeasurementFcn2SampleTime Prompt: Measurement 2
      mask DialogControl MeasurementFcn3SampleTime Prompt: Measurement 3
      mask DialogControl MeasurementFcn4SampleTime Prompt: Measurement 4
      mask DialogControl MeasurementFcn5SampleTime Prompt: Measurement 5
      mask DialogControl ContainerSettings Prompt: shared_tracking:blocks:maskPromptEKFUKFSettings
      mask DialogControl UseCurrentEstimator Prompt: Use the current measurements to improve state estimates
      mask DialogControl OutputStateCovariance Prompt: Output state estimation error covariance
      mask DialogControl DataType Prompt: Data type:
      mask DialogControl SampleTime Prompt: Sample time:
  Extract Diagonal1 : matrix_library/Extract Diagonal
  MATLAB Function : MATLAB Function  TreatAsAtomicUnit=on
  Memory : Memory
  Mux{,1,3..4} (4 alike) : Mux  Inputs=3
  Mux2 : Mux  Inputs=2
  Rate Transition{5..8} (4 alike) : RateTransition  OutPortSampleTime=dt
  Scope{,1..3,5..7} (7 alike) : Scope
  Scope8 : Scope  NumInputPorts=2
  Simulink Function - GPS Measurements : Subsystem  TreatAsAtomicUnit=on
  Simulink Function - GPS Measurements1 : Subsystem  TreatAsAtomicUnit=on
  Simulink Function - GPS Measurements2 : Subsystem  TreatAsAtomicUnit=on
  Simulink Function - GPS Measurements4 : Subsystem  TreatAsAtomicUnit=on
  Simulink Function - State Transition : Subsystem  TreatAsAtomicUnit=on
  Simulink Function - State Transition Jacobian : Subsystem  TreatAsAtomicUnit=on
  Subsystem : Subsystem
  Subsystem1 : Subsystem
  Switch : Switch  Criteria=u2 > Threshold  Threshold=300  SaturateOnIntegerOverflow=off  InputSameDT=off
  Switch2 : Switch  Criteria=u2 > Threshold  Threshold=300  SaturateOnIntegerOverflow=off  InputSameDT=off
  Switch3 : Switch  Criteria=u2 > Threshold  Threshold=300  SaturateOnIntegerOverflow=off  InputSameDT=off
  Terminator : Terminator
  p_r_psi_phi1 : InportShadow  Port=4
  delta_state : Outport
  Measuemrnt Enable Flag : Outport  Port=2
  EKFState : Outport  Port=3
  wires:
  Mux/1 -> Scope3/1, [pos_NED]
  Bus Selector2/2 -> [v_INS]  "<INSstate_v>"
  Data Store Read6/1 -> Scope8/2
  Data Store Read5/1 -> Scope8/1
  Data Type Conversion6/1 -> Extended Kalman Filter1/1(Q)
  Rate Transition5/1 -> Data Type Conversion6/1
  Cal Q1/1(Qd) -> Rate Transition5/1
  Rate Transition8/1 -> Extended Kalman Filter1/4(R1)
  Rate Transition7/1 -> Extended Kalman Filter1/3(y1)
  Rate Transition6/1 -> Extended Kalman Filter1/2(Enable1)
  Extract Diagonal1/1 -> Scope6/1, Bus Creator1/2  "covariance"
  Extended Kalman Filter1/2(P) -> Extract Diagonal1/1
  Subsystem1/1(dp/dv) -> Rate Transition7/1, Scope1/1
  [pos_NED] -> Add1/2
  [p_INS] -> Add1/1
  Constant1/1 -> Rate Transition8/1
  [DCM_b_n] -> Simulink Function - GPS Measurements1/1(DCM_b_n)
  [fbxyz] -> Simulink Function - State Transition Jacobian/3(fbxyz)
  [fbxyz] -> Simulink Function - State Transition/3(fbxyz)
  [wxyz] -> Simulink Function - State Transition Jacobian/2(wxyz)
  [wxyz] -> Simulink Function - State Transition/2(wxyz)
  [DCM_b_n] -> Simulink Function - State Transition Jacobian/1(DCM_b_n)
  [DCM_b_n] -> Simulink Function - State Transition/1(DCM_b_n)
  MATLAB Function/3(dtheta) -> Bus Creator/3  "KFState_dtheta"
  MATLAB Function/1(dp) -> Bus Creator/1  "KFState_dp"
  Extended Kalman Filter1/1(xhat) -> Data Type Conversion1/1, Scope/1
  Subsystem/1(flag) -> Scope5/1, Data Store Write/1
  [pos_NED] -> Subsystem/1(data)
  Data Store Read1/1 -> Scope7/1
  Bus Selector/6 -> Mux1/2  "<ve_gps>"
  Sensor_data/1 -> Bus Selector/1
  Mux1/1 -> Terminator/1, Scope2/1, [vel_NED]
  Bus Selector/5 -> Mux1/1  "<vn_gps>"
  Bus Selector/7 -> Mux1/3  "<vd_gps>"
  Bus Selector/3 -> Mux/2  "<pos_E_gps>"
  Bus Selector/2 -> Mux/1  "<pos_N_gps>"
  Bus Selector/4 -> Mux/3  "<pos_D_gps>"
  Data Store Read4/1 -> Measuemrnt Enable Flag/1
  INS state/1 -> Bus Selector2/1
  Bus Selector2/4 -> [wxyz]  "<INSstate_w>"
  Bus Selector2/5 -> [fbxyz]  "<INSstate_fb>"
  Bus Selector2/1 -> [DCM_b_n]  "<DCM_b_n>"
  Bus Selector2/3 -> Data Type Conversion5/1, [p_INS]  "<INSstste_p>"
  MATLAB Function/4(da) -> Bus Creator/4  "KFState_da"
  MATLAB Function/2(dv) -> Bus Creator/2  "KFState_dv"
  MATLAB Function/5(dg) -> Bus Creator/5  "KFState_dg"
  Data Type Conversion1/1 -> Memory/1
  Bus Creator/1 -> Bus Creator1/1, delta_state/1  "delta_state"
  Memory/1 -> MATLAB Function/1(u)
  Data Store Read3/1 -> Rate Transition6/1, Switch/3
  Add1/1 -> Mux2/1
  Add2/1 -> Mux2/2
  [v_INS] -> Add2/1
  [vel_NED] -> Add2/2
  Bus Creator1/1 -> EKFState/1
  Digital Clock1/1 -> Switch/2
  Constant/1 -> Switch/1
  [pos_NED] -> Switch3/3
  [pos_NED_s2] -> Switch3/1
  Digital Clock/1 -> Switch3/2, Switch2/2
  Switch2/1 -> Subsystem1/2(v_G)
  [v_INS] -> Subsystem1/1(v_I)
  [vel_NED_s2] -> Switch2/1
  [p_INS] -> Subsystem1/3(p_I)
  [vel_NED] -> Switch2/3
  Switch3/1 -> Subsystem1/4(p_G)
  Sensor_data2/1 -> Bus Selector1/1
  Bus Selector1/2 -> Mux3/1  "<pos_N_gps>"
  Bus Selector1/3 -> Mux3/2  "<pos_E_gps>"
  Bus Selector1/4 -> Mux3/3  "<pos_D_gps>"
  Mux3/1 -> [pos_NED_s2]
  Bus Selector1/5 -> Mux4/1  "<vn_gps>"
  Bus Selector1/6 -> Mux4/2  "<ve_gps>"
  Bus Selector1/7 -> Mux4/3  "<vd_gps>"
  Mux4/1 -> [vel_NED_s2]
  p_r_psi_phi/1 -> Bus Selector3/1
  Bus Selector3/1 -> Subsystem1/5(r_k)  "<r12_k>"
  Bus Selector3/3 -> ?  "<dp>"
  Data Type Conversion4/1 -> Simulink Function - GPS Measurements4/2(psi13)
  Data Type Conversion5/1 -> Simulink Function - GPS Measurements4/5(p_INS)
  Data Type Conversion3/1 -> Simulink Function - GPS Measurements4/1(psi12)
  Data Type Conversion8/1 -> Simulink Function - GPS Measurements4/3(p2)
  Data Type Conversion7/1 -> Simulink Function - GPS Measurements4/4(p3)
  p_r_psi_phi1/1 -> Bus Selector4/1
  Bus Selector4/2 -> Data Type Conversion4/1  "<psi12_k-1>"
  Bus Selector4/1 -> Data Type Conversion3/1  "<psi12_k>"
  Bus Selector4/3 -> Data Type Conversion8/1  "<p2>"
  Bus Selector4/4 -> Data Type Conversion7/1  "<p2_k-1>"
  Bus Selector3/5 -> Subsystem1/8(<p2_k-1>)  "<p2_k-1>"
  Bus Selector3/4 -> Subsystem1/7(<p2_k>)  "<p2>"
  Bus Selector3/2 -> Subsystem1/6(r_k-1)  "<r12_k-1>"
  Bus Selector3/6 -> Subsystem1/9(psi_k)  "<psi12_k>"
  Bus Selector3/7 -> Subsystem1/10(psi_k-1)  "<psi12_k-1>"

== system VB_RIFKF_UWB_INS25/ER EKF M1/INS propogation ==
  note: q(1:3)
  Sensor_data : Inport
  Measuemrnt Enable Flag : Inport  Port=2
  delta_state : Inport  Port=3
  Bus Creator : BusCreator  Inputs=7
  Bus Selector : BusSelector  OutputSignals=IMU_Data.gyro_B_rad/s_LPF,IMU_Data.accl_B_m/s2_LPF,MAGN_Data,QGC_sensor_reinit,GPS_Data.pos_N_gps,GPS_Data.pos_E_gps,GPS_Data.pos_D_gps,GPS_Data.vn_gps,GPS_Data.ve_gps,GPS_Data.vd_gps
  Bus Selector1 : BusSelector  OutputSignals=DCM_b_n
  Bus Selector2 : BusSelector  OutputSignals=KFState_dp,KFState_dv,KFState_dtheta,KFState_da,KFState_dg
  Data Type Conversion : DataTypeConversion  OutDataTypeStr=single  SaturateOnIntegerOverflow=off  RndMeth=Floor
  Gain : Gain  Gain=0.1
  Gain1 : Gain  Gain=0.1
  Init_PVQ : Subsystem
  Mux : Mux  Inputs=3
  Mux1 : Mux  Inputs=3
  Scope : Scope  NumInputPorts=2
  accl bias compensation : Subsystem
  att_update : Subsystem
  gyro bias compensation : Subsystem
  vel_pos_update : Subsystem
  INSstate : Outport
  wires:
  Init_PVQ/1(quat_0) -> att_update/3(quat_0)
  [fbxyz] -> vel_pos_update/2(Ab)
  [QGC_init] -> att_update/4(init_flag)
  Bus Selector/10 -> Mux1/3  "<vd_gps>"
  [vel_NED] -> Data Type Conversion/1
  Bus Selector/7 -> Mux/3  "<pos_D_gps>"
  Bus Selector/8 -> Mux1/1  "<vn_gps>"
  Bus Selector/5 -> Mux/1  "<pos_N_gps>"
  [dtheta] -> att_update/1(dtheta)
  [wxyz] -> att_update/2(gyro)
  Bus Selector/6 -> Mux/2  "<pos_E_gps>"
  Bus Selector/3 -> [Magn]  "<MAGN_Data>"
  Mux1/1 -> [vel_NED]
  Sensor_data/1 -> Bus Selector/1
  [fbxyz] -> Init_PVQ/2(accl_B_m/s2_LPF)
  Init_PVQ/2(v0) -> vel_pos_update/3(v0)
  Init_PVQ/3(p0) -> vel_pos_update/4(p0)
  Bus Selector/9 -> Mux1/2  "<ve_gps>"
  [QGC_init] -> vel_pos_update/5(QGC_init)
  [pos_NED] -> Init_PVQ/4(pos_NED)
  Data Type Conversion/1 -> Init_PVQ/5(vel_NED)
  [dp] -> vel_pos_update/6(dp)
  [Magn] -> Init_PVQ/3(Magn_B_guess_LPF)
  Bus Selector/4 -> [QGC_init]  "<QGC_sensor_reinit>"
  Bus Selector/1 -> [gyro_raw]  "<gyro_B_rad/s_LPF>"
  Bus Selector1/1 -> vel_pos_update/1(<DCM_b_n>)  "<DCM_b_n>"
  vel_pos_update/2(V) -> Bus Creator/3  "INSstate_v"
  [dv] -> vel_pos_update/7(dv)
  [QGC_init] -> Init_PVQ/1(QGC_sensor_reinit)
  vel_pos_update/1(p_k) -> Bus Creator/2  "INSstste_p"
  [wxyz] -> Bus Creator/4  "INSstate_w"
  [fbxyz] -> Bus Creator/5  "INSstate_fb"
  att_update/1(att_update) -> Bus Creator/1, Bus Selector1/1  "RotationData"
  Bus Creator/1 -> INSstate/1  "EKF_INSstate"
  accl bias compensation/1(fb) -> Scope/2, [fbxyz]
  accl bias compensation/2(da) -> [da]
  Measuemrnt Enable Flag/1 -> gyro bias compensation/3(Measuemrnt Enable Flag)
  gyro bias compensation/1(wb) -> [wxyz]
  gyro bias compensation/2(dg) -> [dg]
  [dg] -> Bus Creator/6  "INSstate_dg"
  [da] -> Bus Creator/7  "INSstate_da"
  delta_state/1 -> Bus Selector2/1
  Bus Selector2/1 -> [dp]  "<KFState_dp>"
  Bus Selector2/2 -> [dv]  "<KFState_dv>"
  Bus Selector2/3 -> [dtheta]  "<KFState_dtheta>"
  Bus Selector2/4 -> [dda]  "<KFState_da>"
  Bus Selector2/5 -> [ddg]  "<KFState_dg>"
  [gyro_raw] -> gyro bias compensation/1(raw <gyro_B_rad/s_LPF>)
  [accl_raw] -> Scope/1, accl bias compensation/1(raw <accl_B_m/s2_LPF>)
  Bus Selector/2 -> [accl_raw]  "<accl_B_m/s2_LPF>"
  Mux/1 -> [pos_NED]
  [ddg] -> Gain/1
  [dda] -> Gain1/1
  Gain/1 -> gyro bias compensation/2(ddg)
  Gain1/1 -> accl bias compensation/2(dda)
